simulink model "s_torce1"  (Simulink 4.00)
settings: Solver=ode45  SolverMode=SingleTasking  StartTime=0.0  StopTime=200  MaxStep=0.1  RelTol=1e-3  AbsTol=1e-6
values from neighbouring files (symbols this model uses):
  A1 = 2    [torce11.m]    (also in torcell.mat; waag11.mat)
  A12 = 0.1    [torce11.m]    (also in torcell.mat; waag11.mat)
  A2 = 2    [torce11.m]    (also in torcell.mat; waag11.mat)
  g = 9.8    [ident21.mat]    (also in torce11.m = 9.81; torcell.mat = 9.81; waag11.m = 9.81; waag11.mat = 9.81)
settings Model: LastModifiedBy=Administrator  SaveTime=off  SaveOutput=off  LimitDataPoints=off  BlockReductionOpt=off

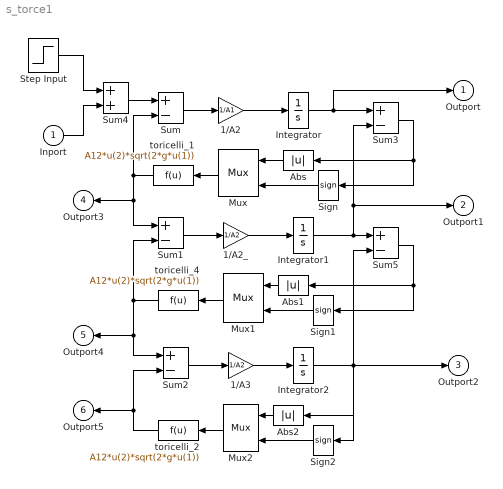
== system s_torce1 ==
  Inport : Inport  Port=1
  1/A2 : Gain  Gain=1/A1  Multiplication=Element-wise(K.*u)  SaturateOnIntegerOverflow=on
  1/A2_ : Gain  Gain=1/A2  Multiplication=Element-wise(K.*u)  SaturateOnIntegerOverflow=on
  1/A3 : Gain  Gain=1/A2  Multiplication=Element-wise(K.*u)  SaturateOnIntegerOverflow=on
  Abs : Abs  Orientation=left  SaturateOnIntegerOverflow=on
  Abs1 : Abs  Orientation=left  SaturateOnIntegerOverflow=on
  Abs2 : Abs  Orientation=left  SaturateOnIntegerOverflow=on
  Integrator : Integrator  ExternalReset=none  InitialConditionSource=internal  InitialCondition=0  LimitOutput=off  UpperSaturationLimit=inf  LowerSaturationLimit=-inf  ShowSaturationPort=off  ShowStatePort=off  AbsoluteTolerance=auto
  Integrator1 : Integrator  ExternalReset=none  InitialConditionSource=internal  InitialCondition=0  LimitOutput=off  UpperSaturationLimit=inf  LowerSaturationLimit=-inf  ShowSaturationPort=off  ShowStatePort=off  AbsoluteTolerance=auto
  Integrator2 : Integrator  ExternalReset=none  InitialConditionSource=internal  InitialCondition=0  LimitOutput=off  UpperSaturationLimit=inf  LowerSaturationLimit=-inf  ShowSaturationPort=off  ShowStatePort=off  AbsoluteTolerance=auto
  Mux : Mux  Orientation=left  Inputs=2
      settings: DisplayOption=none
  Mux1 : Mux  Orientation=left  Inputs=2
      settings: DisplayOption=none
  Mux2 : Mux  Orientation=left  Inputs=2
      settings: DisplayOption=none
  Sign : Signum  Orientation=left
  Sign1 : Signum  Orientation=left
  Sign2 : Signum  Orientation=left
  Step Input : Step  Time=0  Before=0  After=1  SampleTime=0
  Sum{,1..3,5} (5 alike) : Sum  Inputs=+-  SaturateOnIntegerOverflow=on
  Sum4 : Sum  Inputs=++  SaturateOnIntegerOverflow=on
  toricelli_1 : Fcn  Orientation=left  Expr=A12*u(2)*sqrt(2*g*u(1))
  toricelli_2 : Fcn  Orientation=left  Expr=A12*u(2)*sqrt(2*g*u(1))
  toricelli_4 : Fcn  Orientation=left  Expr=A12*u(2)*sqrt(2*g*u(1))
  Outport : Outport  Port=1
  Outport1 : Outport  Port=2
  Outport2 : Outport  Port=3
  Outport3 : Outport  Orientation=left  Port=4
  Outport4 : Outport  Orientation=left  Port=5
  Outport5 : Outport  Orientation=left  Port=6
  wires:
  Inport/1 -> Sum4/2
  Step Input/1 -> Sum4/1
  Sum4/1 -> Sum/1
  toricelli_2/1 -> Outport5/1, Sum2/2
  Integrator/1 -> Outport/1, Sum3/1
  Integrator2/1 -> Sign2/1, Outport2/1, Abs2/1, Sum5/2
  Sign2/1 -> Mux2/2
  Mux2/1 -> toricelli_2/1
  Abs2/1 -> Mux2/1
  toricelli_4/1 -> Outport4/1, Sum2/1, Sum1/2
  Abs1/1 -> Mux1/1
  Sum5/1 -> Abs1/1, Sign1/1
  Sign1/1 -> Mux1/2
  Mux1/1 -> toricelli_4/1
  Sign/1 -> Mux/2
  Mux/1 -> toricelli_1/1
  Abs/1 -> Mux/1
  Sum3/1 -> Sign/1, Abs/1
  toricelli_1/1 -> Outport3/1, Sum1/1, Sum/2
  Integrator1/1 -> Outport1/1, Sum3/2, Sum5/1
  1/A3/1 -> Integrator2/1
  1/A2_/1 -> Integrator1/1
  1/A2/1 -> Integrator/1
  Sum2/1 -> 1/A3/1
  Sum1/1 -> 1/A2_/1
  Sum/1 -> 1/A2/1
